simulink model "M_FOC"  (R2022a)
settings: Solver=FixedStepAuto  StartTime=0.0  StopTime=2  FixedStep=1e-6  RelTol=1e-3
libraries: simulink x1
settings Model: Creator=Mengyang  LastModifiedBy=Mengyang

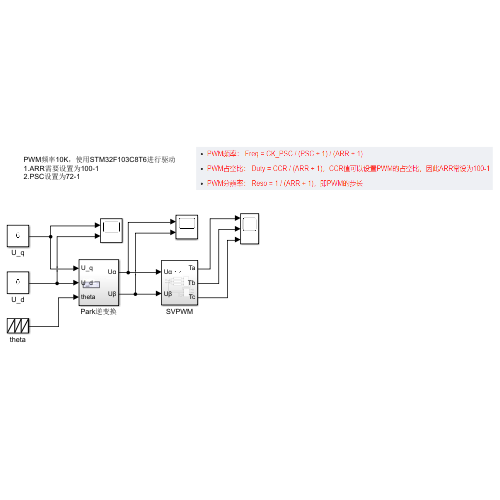
[thumbnail: Simulink's stored preview of the top-level diagram]
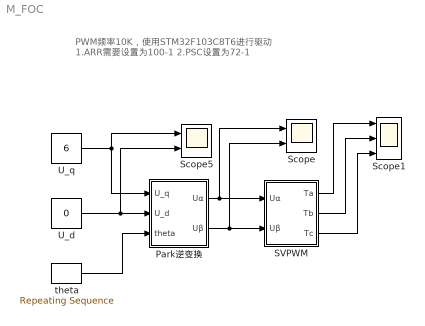
== system M_FOC ==
  note: PWM频率10K，使用STM32F103C8T6进行驱动
      | 1.ARR需要设置为100-1
      | 2.PSC设置为72-1
  Park逆变换 : Subsystem
  SVPWM : Subsystem
  Scope : Scope  NumInputPorts=2
  Scope1 : Scope  NumInputPorts=3
  Scope5 : Scope  NumInputPorts=2
  U_d : Constant  Value=0
  U_q : Constant  Value=6
  "theta " : simulink/Sources/Repeating Sequence  rep_seq_t=[0 1]  rep_seq_y=[0 2*pi]
  wires:
  U_q/1 -> Scope5/1, Park逆变换/1(U_q)
  U_d/1 -> Scope5/2, Park逆变换/2(U_d)
  "theta "/1 -> Park逆变换/3(theta)
  Park逆变换/1(Uα) -> Scope/1, SVPWM/1(Uα)
  Park逆变换/2(Uβ) -> Scope/2, SVPWM/2(Uβ)
  SVPWM/1(Ta) -> Scope1/1
  SVPWM/2(Tb) -> Scope1/2
  SVPWM/3(Tc) -> Scope1/3

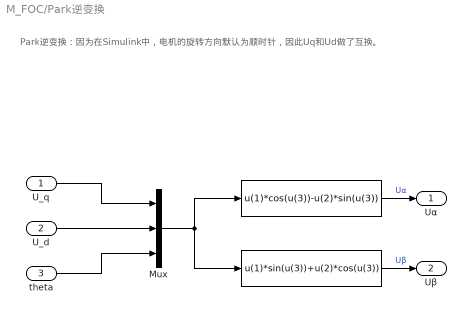
== system M_FOC/Park逆变换 ==
  note: Park逆变换：因为在Simulink中，电机的旋转方向默认为顺时针，因此Uq和Ud做了互换。
  U_q : Inport
  U_d : Inport  Port=2
  theta : Inport  Port=3
  " " : Fcn  Expr=u(1)*cos(u(3))-u(2)*sin(u(3))
  "  " : Fcn  Expr=u(1)*sin(u(3))+u(2)*cos(u(3))
  Mux : Mux  Inputs=3
  Uα : Outport
  Uβ : Outport  Port=2
  wires:
  Mux/1 -> "  "/1, " "/1
  theta/1 -> Mux/3
  U_d/1 -> Mux/2
  "  "/1 -> Uβ/1  "Uβ"
  " "/1 -> Uα/1  "Uα"
  U_q/1 -> Mux/1

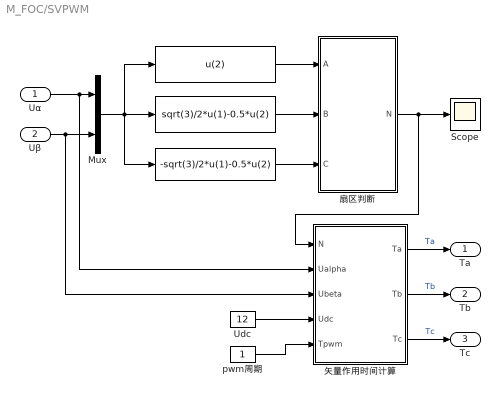
== system M_FOC/SVPWM ==
  Uα : Inport
  Uβ : Inport  Port=2
  " " : Fcn  Expr=u(2)
  "  " : Fcn  Expr=sqrt(3)/2*u(1)-0.5*u(2)
  "   " : Fcn  Expr=-sqrt(3)/2*u(1)-0.5*u(2)
  Mux : Mux  Inputs=2
  Scope : Scope
  Udc : Constant  Value=12
  pwm周期 : Constant
  扇区判断 : MATLAB Function  TreatAsAtomicUnit=on
  矢量作用时间计算 : MATLAB Function  TreatAsAtomicUnit=on
  Ta : Outport
  Tb : Outport  Port=2
  Tc : Outport  Port=3
  wires:
  Uα/1 -> 矢量作用时间计算/2(Ualpha), Mux/1
  Uβ/1 -> 矢量作用时间计算/3(Ubeta), Mux/2
  Mux/1 -> " "/1, "   "/1, "  "/1
  " "/1 -> 扇区判断/1(A)
  "  "/1 -> 扇区判断/2(B)
  "   "/1 -> 扇区判断/3(C)
  扇区判断/1(N) -> 矢量作用时间计算/1(N), Scope/1
  矢量作用时间计算/1(Ta) -> Ta/1  "Ta"
  矢量作用时间计算/2(Tb) -> Tb/1  "Tb"
  矢量作用时间计算/3(Tc) -> Tc/1  "Tc"
  Udc/1 -> 矢量作用时间计算/4(Udc)
  pwm周期/1 -> 矢量作用时间计算/5(Tpwm)

== matlab function M_FOC/SVPWM/扇区判断 ==
  data: A input; N output; B input; C input
function N = SectorJudge(A,B,C)
N=0;

% N = A + 2B + 4C
if(A>0)
    N=N+1;
end

if(B>0)
    N=N+2;
end

if(C>0)
    N=N+4;
end

== matlab function M_FOC/SVPWM/矢量作用时间计算 ==
  data: N input; Ta output; Ualpha input; Ubeta input; Udc input; Tpwm input; Tb output; Tc output
function [Ta,Tb,Tc] = VectorCalculate(N,Ualpha,Ubeta,Udc,Tpwm)

Ta=double(0);
Tb=double(0);
Tc=double(0);

M = sqrt(3)*Tpwm/Udc;
U1 = Ubeta*M;
U2 = (sqrt(3)*Ualpha/2 - 0.5 * Ubeta)*M;
U3 = (-sqrt(3)*Ualpha/2 - 0.5 * Ubeta)*M;

%% 扇区1
if(N==3)  
   T4 = U2;
   T6 = U1;
   SUM = T4+T6;
   if(SUM>Tpwm)
       K_SVPWM = Tpwm/SUM;
       T4= K_SVPWM*T4;
       T6= K_SVPWM*T6;
   end
   T7=(Tpwm-T4-T6)/2;
   Ta = T4+T6+T7;
   Tb = T6+T7;
   Tc = T7;
end
%% 扇区2
if(N==1)  
   T2 = -U2;
   T6 = -U3;
   SUM = T2+T6;
   if(SUM>Tpwm)
       K_SVPWM = Tpwm/SUM;
       T2= K_SVPWM*T2;
       T6= K_SVPWM*T6;
   end
   T7=(Tpwm-T2-T6)/2;
   Ta = T6+T7;
   Tb = T2+T6+T7;
   Tc = T7;
end
%% 扇区3
if(N==5)  
   T2 = U1;
   T3 = U3;
   SUM = T2+T3;
   if(SUM>Tpwm)
       K_SVPWM = Tpwm/SUM;
       T2= K_SVPWM*T2;
       T3= K_SVPWM*T3;
   end
   T7=(Tpwm-T2-T3)/2;
   Ta = T7;
   Tb = T2+T3+T7;
   Tc = T3+T7;
end
%% 扇区4
if(N==4)  
   T1 = -U1;
   T3 = -U2;
   SUM = T1+T3;
   if(SUM>Tpwm)
       K_SVPWM = Tpwm/SUM;
       T1= K_SVPWM*T1;
       T3= K_SVPWM*T3;
   end
   T7=(Tpwm-T1-T3)/2;
   Ta = T7;
   Tb = T3+T7;
   Tc = T1+T3+T7;
end
%% 扇区5
if(N==6)  
   T1 = U3;
   T5 = U2;
   SUM = T1+T5;
   if(SUM>Tpwm)
       K_SVPWM = Tpwm/SUM;
       T1= K_SVPWM*T1;
       T5= K_SVPWM*T5;
   end
   T7=(Tpwm-T1-T5)/2;
   Ta = T5+T7;
   Tb = T7;
   Tc = T1+T5+T7;
end
%% 扇区6
if(N==2)  
   T4 = -U3;
   T5 = -U1;
   SUM = T4+T5;
   if(SUM>Tpwm)
       K_SVPWM = Tpwm/SUM;
       T4= K_SVPWM*T4;
       T5= K_SVPWM*T5;
   end
   T7=(Tpwm-T4-T5)/2;
   Ta = T4+T5+T7;
   Tb = T7;
   Tc = T5+T7;
end
